simulink model "bldc_model"  (R2016a)
settings: Solver=ode45  StartTime=0.0  StopTime=1  RelTol=1e-3
values from neighbouring files (symbols this model uses):
  Dm = 6.04e-6    (= 6.04e-06)    [init_params_BLDC.m]
  J = 2.12e-6    (= 2.12e-06)    [init_params_BLDC.m]
  Lam = 1.65e-2    (= 0.0165)    [init_params_BLDC.m]
  Lss = 10.1e-3    (= 0.0101)    [init_params_BLDC.m]
  P = 4    [init_params_BLDC.m]
  rs = 5.2    [init_params_BLDC.m]
  Tm = 3.53e-3    (= 0.00353)    [init_params_BLDC.m]
  Ts = Lss/rs    (= 0.00194230769231)    [init_params_BLDC.m]
  Vdc = 6    [init_params_BLDC.m]
settings Model: Creator=Atif Ali  LastModifiedBy=asali
settings DataIOCC: LimitDataPoints=on  SaveFormat=Array
settings HardwareCC: ProdBitPerPointer=32  ProdLargestAtomicFloat=None  ProdIntDivRoundTo=Undefined  ProdEndianess=Unspecified  ProdWordSize=32  ProdHWDeviceType=32-bit Generic
settings ModelReferenceCC: PropagateSignalLabelsOutOfModel=off
settings ConfigComp: CovModelRefEnable=Off

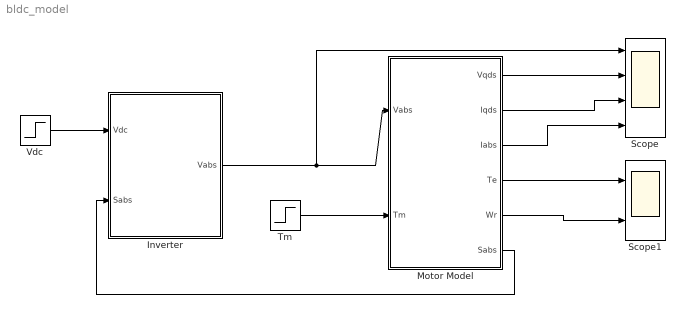
== system bldc_model ==
  Inverter : Subsystem
  Motor Model : Subsystem
  Scope : Scope  NumInputPorts=4
  Scope1 : Scope  NumInputPorts=2
  Tm : Step  Time=0.5  After=Tm  SampleTime=0
  Vdc : Step  Time=0.05  After=Vdc  SampleTime=0
  wires:
  Motor Model/6(Sabs) -> Inverter/2(Sabs)
  Inverter/1(Vabs) -> Scope/1, Motor Model/1(Vabs)
  Tm/1 -> Motor Model/2(Tm)
  Vdc/1 -> Inverter/1(Vdc)
  Motor Model/1(Vqds) -> Scope/2
  Motor Model/2(Iqds) -> Scope/3
  Motor Model/3(Iabs) -> Scope/4
  Motor Model/4(Te) -> Scope1/1
  Motor Model/5(Wr) -> Scope1/2

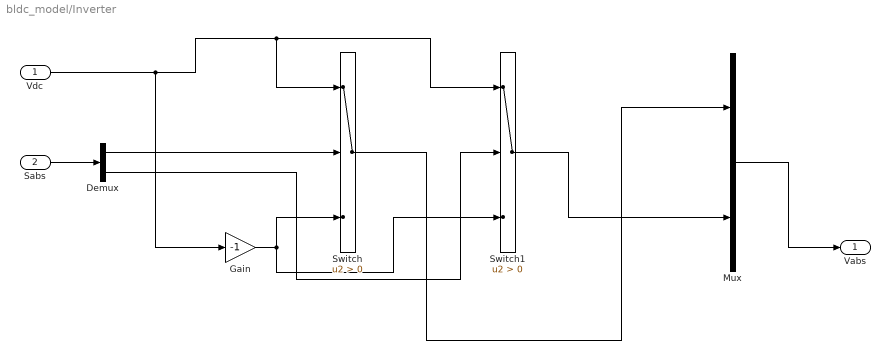
== system bldc_model/Inverter ==
  Vdc : Inport
  Sabs : Inport  Port=2
  Demux : Demux  Outputs=2
  Gain : Gain  Gain=-1
  Mux : Mux  Inputs=2
  Switch : Switch  Criteria=u2 > Threshold
  Switch1 : Switch  Criteria=u2 > Threshold
  Vabs : Outport
  wires:
  Sabs/1 -> Demux/1
  Mux/1 -> Vabs/1
  Demux/1 -> Switch/2
  Vdc/1 -> Gain/1, Switch/1, Switch1/1
  Switch/1 -> Mux/1
  Switch1/1 -> Mux/2
  Demux/2 -> Switch1/2
  Gain/1 -> Switch/3, Switch1/3

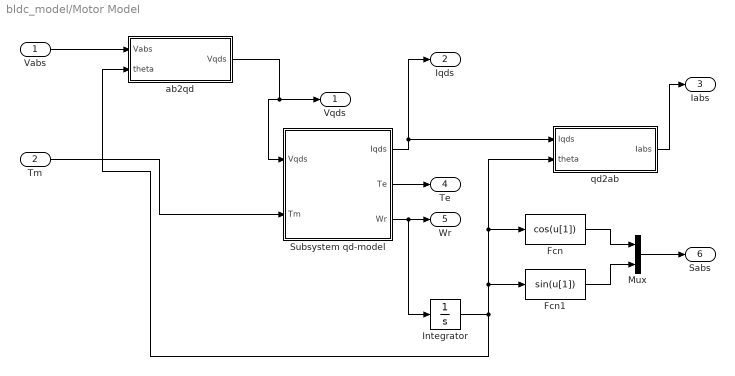
== system bldc_model/Motor Model ==
  Vabs : Inport
  Tm : Inport  Port=2
  Fcn : Fcn  Expr=cos(u[1])
  Fcn1 : Fcn
  Integrator : Integrator
  Mux : Mux  Inputs=2
  Subsystem qd-model : Subsystem
  ab2qd : Subsystem
  qd2ab : Subsystem
  Vqds : Outport
  Iqds : Outport  Port=2
  Iabs : Outport  Port=3
  Te : Outport  Port=4
  Wr : Outport  Port=5
  Sabs : Outport  Port=6
  wires:
  Vabs/1 -> ab2qd/1(Vabs)
  ab2qd/1(" Vqds") -> Subsystem qd-model/1(Vqds), Vqds/1
  Tm/1 -> Subsystem qd-model/2(Tm)
  Subsystem qd-model/1(Iqds) -> Iqds/1, qd2ab/1(Iqds)
  qd2ab/1(" Iabs") -> Iabs/1
  Subsystem qd-model/2(Te) -> Te/1
  Subsystem qd-model/3(Wr) -> Integrator/1, Wr/1
  Integrator/1 -> ab2qd/2(theta), Fcn1/1, qd2ab/2(theta), Fcn/1
  Mux/1 -> Sabs/1
  Fcn/1 -> Mux/1
  Fcn1/1 -> Mux/2

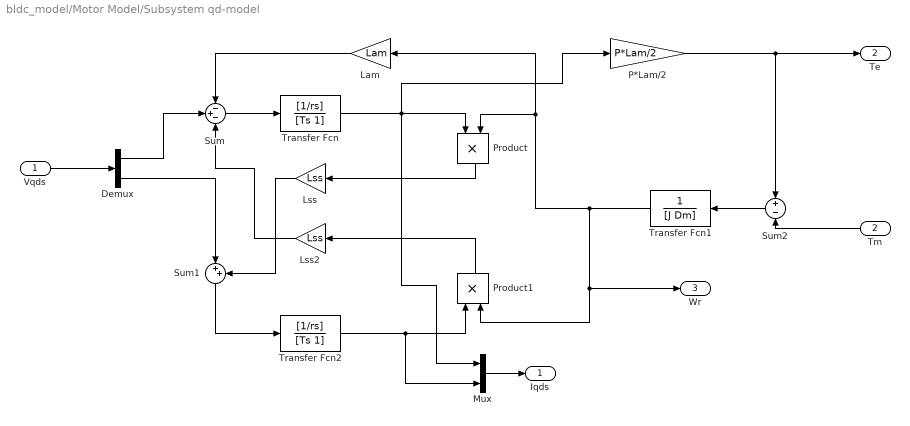
== system bldc_model/Motor Model/Subsystem qd-model ==
  Vqds : Inport
  Tm : Inport  Port=2
  Demux : Demux  Outputs=2
  Lam : Gain  Gain=Lam
  Lss : Gain  Gain=Lss
  Lss2 : Gain  Gain=Lss
  Mux : Mux  Inputs=2
  P*Lam/2 : Gain  Gain=P*Lam/2
  Product : Product
  Product1 : Product
  Sum : Sum  Inputs=-+-
  Sum1 : Sum  Inputs=|++
  Sum2 : Sum  Inputs=+-
  Transfer Fcn : TransferFcn  Numerator=[1/rs]  Denominator=[Ts 1]
  Transfer Fcn1 : TransferFcn  Denominator=[J Dm]
  Transfer Fcn2 : TransferFcn  Numerator=[1/rs]  Denominator=[Ts 1]
  Iqds : Outport
  Te : Outport  Port=2
  Wr : Outport  Port=3
  wires:
  Vqds/1 -> Demux/1
  Demux/1 -> Sum/2
  Demux/2 -> Sum1/1
  P*Lam/2/1 -> Sum2/1, Te/1
  Tm/1 -> Sum2/2
  Sum/1 -> Transfer Fcn/1
  Lam/1 -> Sum/1
  Lss2/1 -> Sum/3
  Lss/1 -> Sum1/2
  Sum1/1 -> Transfer Fcn2/1
  Sum2/1 -> Transfer Fcn1/1
  Transfer Fcn2/1 -> Mux/2, Product1/1
  Product1/1 -> Lss2/1
  Product/1 -> Lss/1
  Transfer Fcn/1 -> Mux/1, P*Lam/2/1, Product/1
  Transfer Fcn1/1 -> Product/2, Lam/1, Product1/2, Wr/1
  Mux/1 -> Iqds/1

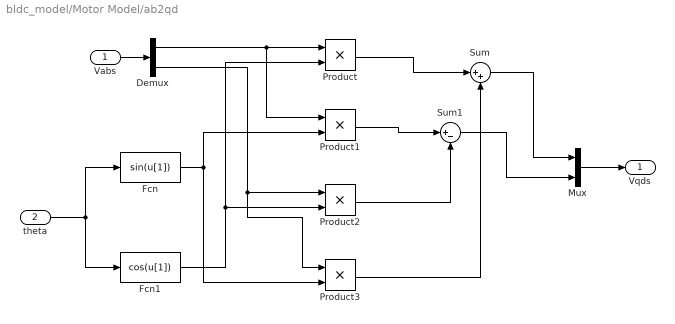
== system bldc_model/Motor Model/ab2qd ==
  Vabs : Inport
  theta : Inport  Port=2
  Demux : Demux  Outputs=2
  Fcn : Fcn
  Fcn1 : Fcn  Expr=cos(u[1])
  Mux : Mux  Inputs=2
  Product{,1..3} (4 alike) : Product
  Sum : Sum  Inputs=|++
  Sum1 : Sum  Inputs=|+-
  " Vqds" : Outport
  wires:
  Vabs/1 -> Demux/1
  Mux/1 -> " Vqds"/1
  theta/1 -> Fcn/1, Fcn1/1
  Demux/1 -> Product1/1, Product/1
  Fcn1/1 -> Product2/2, Product/2
  Fcn/1 -> Product1/2, Product3/2
  Demux/2 -> Product3/1, Product2/1
  Product/1 -> Sum/1
  Product3/1 -> Sum/2
  Sum/1 -> Mux/1
  Product1/1 -> Sum1/1
  Product2/1 -> Sum1/2
  Sum1/1 -> Mux/2

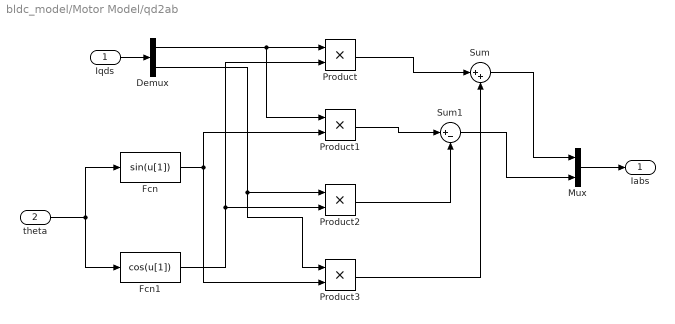
== system bldc_model/Motor Model/qd2ab ==
  Iqds : Inport
  theta : Inport  Port=2
  Demux : Demux  Outputs=2
  Fcn : Fcn
  Fcn1 : Fcn  Expr=cos(u[1])
  Mux : Mux  Inputs=2
  Product{,1..3} (4 alike) : Product
  Sum : Sum  Inputs=|++
  Sum1 : Sum  Inputs=|+-
  " Iabs" : Outport
  wires:
  Iqds/1 -> Demux/1
  Mux/1 -> " Iabs"/1
  theta/1 -> Fcn/1, Fcn1/1
  Demux/1 -> Product1/1, Product/1
  Fcn1/1 -> Product2/2, Product/2
  Fcn/1 -> Product1/2, Product3/2
  Demux/2 -> Product3/1, Product2/1
  Product/1 -> Sum/1
  Product3/1 -> Sum/2
  Sum/1 -> Mux/1
  Product1/1 -> Sum1/1
  Product2/1 -> Sum1/2
  Sum1/1 -> Mux/2
